simulink model "inv_M_2x2"  (R2017b)
settings: Solver=FixedStepDiscrete  StartTime=0.0  StopTime=19.8  FixedStep=0.200000  MaxStep=.2  RelTol=1e-3  EnableMultiTasking=on
model workspace (MAT data in the model file):
  Var = 0
  already_pp = 0
  input_struct.time = [0; 0.2; 0.4; 0.6; 0.8; 1; 1.2; 1.4; 1.6; 1.8; 2; 2.2; 2.4; 2.6; 2.8; 3; 3.2; 3.4; 3.6; 3.8; 4; 4.2; 4.4; 4.6; 4.8; 5; 5.2; 5.4; 5.6; 5.8; 6; 6.2; 6.4; 6.6; 6.8; 7; 7.2; 7.4; 7.6; 7.8; 8; 8.2; 8.4; 8.6; 8.8; 9; 9.2; 9.4; 9.6; 9.8; 10; 10.2; 10.4; 10.6; 10.8; 11; 11.2; 11.4; 11.6; 11.8; 12; 12.2; 12.4; 12.6; 12.8; 13; 13.2; 13.4; 13.6; 13.8; 14; 14.2; 14.4; 14.6; 14.8; 15; 15.2; 15.4; 15.6; 15.8; 16; 16.2; 16.4; 16.6; 16.8; 17; 17.2; 17.4; 17.6; 17.8; 18; 18.2; 18.4; 18.6; 18.8; 19; 19.2; 19.4; 19.6; 19.8]
  input_struct.signals(1).name = 'A'
  input_struct.signals(1).values = [-172.344593938 -251.025974973 -135.312355269 220.51103188 35.6142404385 -21.2233373836 -41.8194595318 164.391552012 92.3522527685 94.6375629999 -203.387457249 -40.5739038338 ... (400 elements, 2x2x100)]
  input_struct.signals(1).dimensions = [2 2]
  input_struct.signals(2).name = 'B'
  input_struct.signals(2).values = [-299.86136088 -210.321760579 -135.699419073 223.455011378 60.7506863471 -107.286928301 -129.424155326 -38.8105165295 242.255430709 255.063386992 3.1754713235 76.549085562 ... (400 elements, 2x2x100)]
  input_struct.signals(2).dimensions = [2 2]
  input_struct.signals(3).name = 'C'
  input_struct.signals(3).values = [228.503476476 -131.589109443 59.4855055852 -284.264316811 -206.880800239 200.34652243 -183.06397965 197.872821062 -97.1550845823 102.669929719 -268.580208562 140.585439831 ... (400 elements, 2x2x100)]
  input_struct.signals(3).dimensions = [2 2]
settings Model: Creator=ktrinh  LastModifiedBy=hbourbou
settings DataIOCC: ExternalInput=input_struct  LoadExternalInput=on  SaveFormat=Structure  SaveState=on
settings OptimizationCC: LifeSpan=inf
settings DebuggingCC: AlgebraicLoopMsg=error  ArtificialAlgebraicLoopMsg=error  SFUnexpectedBacktrackingDiag=warning  SFNoUnconditionalDefaultTransitionDiag=warning  SFExecutionAtInitializationDiag=none
settings HardwareCC: ProdBitPerSizeT=32  ProdBitPerPtrDiffT=32  ProdWordSize=32  ProdHWDeviceType=Specified
settings CodeAppCC: StateflowObjectComments=on
settings GRTTargetCC: TargetLangStandard=C89/C90 (ANSI)  GeneratePreprocessorConditionals=Disable all  ExtMode=on
settings ConfigComp: CovMetricSettings=dw  CovHtmlReporting=on  CovSaveCumulativeToWorkspaceVar=on  CovSaveSingleToWorkspaceVar=on  CovExternalEMLEnable=off

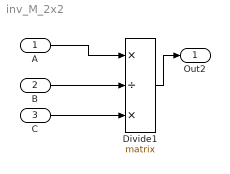
== system inv_M_2x2 ==
  A : Inport  OutDataTypeStr=double  PortDimensions=[2 2]
  B : Inport  Port=2  OutDataTypeStr=double  PortDimensions=[2 2]
  C : Inport  Port=3  OutDataTypeStr=double  PortDimensions=[2 2]
  Divide1 : Product  Inputs=*/*  Multiplication=Matrix(*)
  Out2 : Outport
  wires:
  Divide1/1 -> Out2/1
  A/1 -> Divide1/1
  B/1 -> Divide1/2
  C/1 -> Divide1/3
